simulink model "gm_Image_threshold_final"  (R2018b)
settings: Solver=FixedStepAuto  StartTime=0.0  StopTime=10.0  RelTol=1e-3  EnableMultiTasking=on
libraries: visionsources x1, dspmtrx3 x1
settings Model: Creator=Administrator  LastModifiedBy=Administrator
settings SolverCC: AutoInsertRateTranBlk=on
settings OptimizationCC: BlockReduction=off  ConditionallyExecuteInputs=off  DefaultParameterBehavior=Inlined
settings DebuggingCC: AlgebraicLoopMsg=error  InheritedTsInSrcMsg=none  SingleTaskRateTransMsg=error
settings HardwareCC: ProdBitPerPointer=32  ProdBitPerSizeT=32  ProdBitPerPtrDiffT=32  ProdLargestAtomicFloat=None  ProdIntDivRoundTo=Undefined  ProdEndianess=Unspecified  ProdWordSize=32  ProdHWDeviceType=ASIC/FPGA->ASIC/FPGA  TargetBitPerPointer=64  TargetBitPerSizeT=64  TargetBitPerPtrDiffT=64  TargetLongLongMode=on  TargetIntDivRoundTo=Zero  TargetEndianess=LittleEndian  TargetWordSize=64  TargetHWDeviceType=Custom Processor->MATLAB Host Computer  ProdEqTarget=off

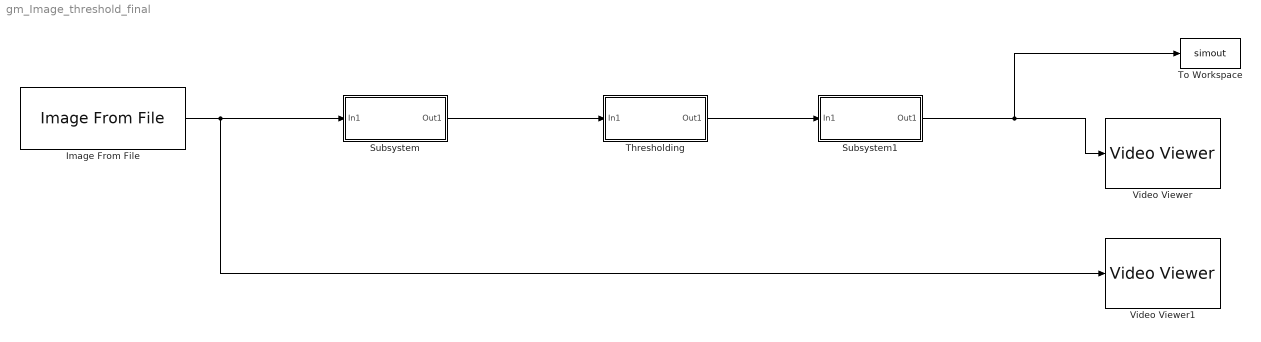
== system gm_Image_threshold_final ==
  Image From File : visionsources/Image From File  Tag=vipblks_nd  FileName=C:\Users\Administrator\Desktop\chapter\101_4.tif  imagePorts=One multidimensional signal  Ts=0.1  ImageDataType=uint8  Signed=on  WordLength=16  sdImageDataType=uint(8)  FractionLengthMode=User-defined  FractionLength=15  OutPortLabels=R|G|B
      settings: SourceProductName=Computer Vision System Toolbox
  Subsystem : Subsystem
  Subsystem1 : Subsystem
  Thresholding : Subsystem  TreatAsAtomicUnit=on
  To Workspace : ToWorkspace  VariableName=simout  SampleTime=-1
      settings: Save2DSignal=2-D array (concatenate along first dimension)
  Video Viewer : VideoViewer  FigPos=[1249 575 418 304]
  Video Viewer1 : VideoViewer  FigPos=[487 497 457 372]
  wires:
  Thresholding/1(Out1) -> Subsystem1/1(In1)
  Subsystem/1(Out1) -> Thresholding/1(In1)
  Image From File/1 -> Subsystem/1(In1), Video Viewer1/1
  Subsystem1/1(Out1) -> Video Viewer/1, To Workspace/1

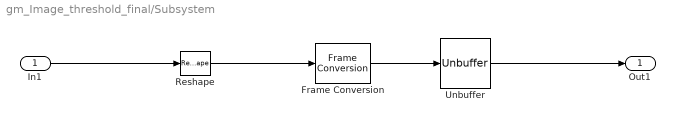
== system gm_Image_threshold_final/Subsystem ==
  In1 : Inport
  Frame Conversion : FrameConversion
  Reshape : Reshape
  Unbuffer : Unbuffer
  Out1 : Outport
  wires:
  In1/1 -> Reshape/1
  Reshape/1 -> Frame Conversion/1
  Unbuffer/1 -> Out1/1
  Frame Conversion/1 -> Unbuffer/1

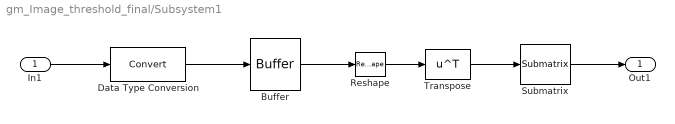
== system gm_Image_threshold_final/Subsystem1 ==
  In1 : Inport
  Buffer : Buffer  N=65536  OutputFrames=off
  Data Type Conversion : DataTypeConversion
  Reshape : Reshape  OutputDimensionality=Customize  OutputDimensions=[256,256]
  Submatrix : dspmtrx3/Submatrix  RowSpan=Range of rows  RowStartMode=First  RowStartIndex=1  RowEndMode=Last  RowEndIndex=1  ColSpan=Range of columns  ColStartMode=First  ColStartIndex=1  ColEndMode=Last  ColEndIndex=1
  Transpose : Math  Operator=transpose  RndMeth=Zero  SaturateOnIntegerOverflow=on
  Out1 : Outport
  wires:
  In1/1 -> Data Type Conversion/1
  Submatrix/1 -> Out1/1
  Transpose/1 -> Submatrix/1
  Reshape/1 -> Transpose/1
  Buffer/1 -> Reshape/1
  Data Type Conversion/1 -> Buffer/1

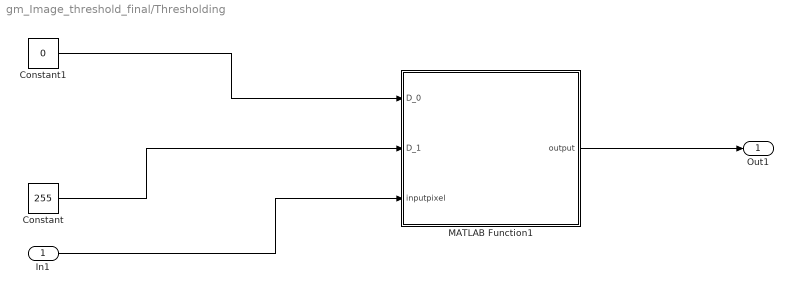
== system gm_Image_threshold_final/Thresholding ==
  In1 : Inport  OutDataTypeStr=uint8  PortDimensions=1  SampleTime=1.52587890625e-06
  Constant : Constant  Value=255  OutDataTypeStr=uint32  SampleTime=-1
  Constant1 : Constant  Value=0  OutDataTypeStr=uint32  SampleTime=-1
  MATLAB Function1 : MATLAB Function  TreatAsAtomicUnit=on
  Out1 : Outport
  wires:
  In1/1 -> MATLAB Function1/3(inputpixel)
  Constant/1 -> MATLAB Function1/2(D_1)
  Constant1/1 -> MATLAB Function1/1(D_0)
  MATLAB Function1/1(output) -> Out1/1

== matlab function gm_Image_threshold_final/Thresholding/MATLAB Function1 ==
  data: D_0 input; output output; D_1 input; inputpixel input
function output = my_new_2_isto_1_mux(D_0,D_1,inputpixel)
if(inputpixel<=120) 
output=D_0; 
else 
output=D_1; 
end 
end
